simulink model "water_tank_pi_with_delay"  (R2024b)
settings: Solver=ode4  StartTime=0.0  StopTime=50  FixedStep=0.001  RelTol=1e-3
libraries: SignalEditorBlockLib x2
settings Model: Creator=max  LastModifiedBy=max

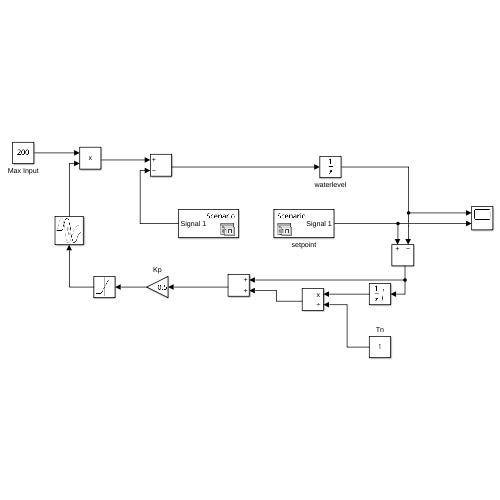
[thumbnail: Simulink's stored preview of the top-level diagram]
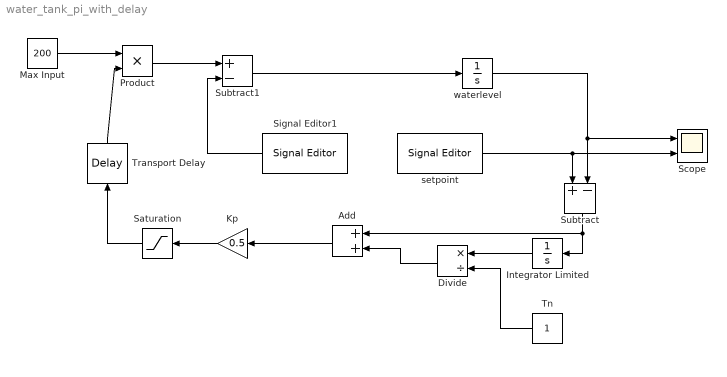
== system water_tank_pi_with_delay ==
  Add : Sum
  Divide : Product  Inputs=*/
  Integrator Limited : Integrator  LimitOutput=on  UpperSaturationLimit=1  LowerSaturationLimit=0
  Kp : Gain  Gain=0.5
  Max Input : Constant  Value=200
  Product : Product
  Saturation : Saturate  UpperLimit=1  LowerLimit=0
  Scope : Scope  NumInputPorts=2
  Signal Editor1 : SignalEditorBlockLib/Signal Editor  FileName=water_loss.mat  ActiveScenario=Scenario  ActiveSignal=Signal 1  IsBus=off  OutputBusObjectStr=Bus: BusObject  SampleTime=0  Interpolate=off  ZeroCross=off  OutputAfterFinalValue=Setting to zero  Unit=inherit  PreserveSignalName=on  ApplySigPropsToAllScenarios=on  ApplySigPropsToAllSignals=off
  Subtract : Sum  Inputs=+-
  Subtract1 : Sum  Inputs=+-
  Tn : Constant
  Transport Delay : TransportDelay  DelayTime=5
  setpoint : SignalEditorBlockLib/Signal Editor  FileName=water_setpoint.mat  ActiveScenario=Scenario  ActiveSignal=Signal 1  IsBus=off  OutputBusObjectStr=Bus: BusObject  SampleTime=0  Interpolate=off  ZeroCross=off  OutputAfterFinalValue=Setting to zero  Unit=inherit  PreserveSignalName=on  ApplySigPropsToAllScenarios=on  ApplySigPropsToAllSignals=off
  waterlevel : Integrator  InitialCondition=1000
  wires:
  waterlevel/1 -> Subtract/2, Scope/1
  setpoint/1 -> Scope/2, Subtract/1
  Integrator Limited/1 -> Divide/1
  Tn/1 -> Divide/2
  Subtract/1 -> Integrator Limited/1, Add/1
  Divide/1 -> Add/2
  Add/1 -> Kp/1
  Kp/1 -> Saturation/1
  Max Input/1 -> Product/1
  Saturation/1 -> Transport Delay/1
  Signal Editor1/1 -> Subtract1/2
  Product/1 -> Subtract1/1
  Subtract1/1 -> waterlevel/1
  Transport Delay/1 -> Product/2
